simulink model "lab2_1"  (R2025b)
settings: Solver=VariableStepAuto  StartTime=0.0  StopTime=25.0  RelTol=1e-3
settings Model: Creator=mizula  LastModifiedBy=mizula

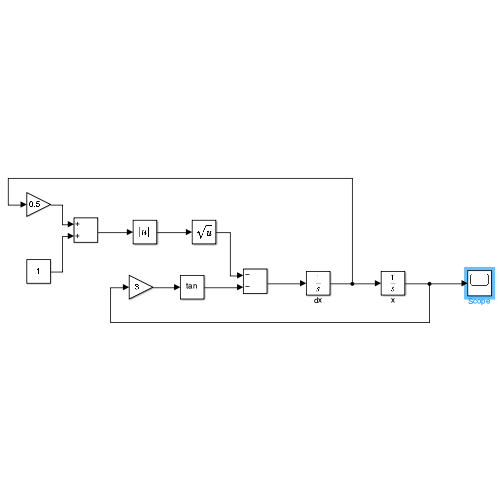
[thumbnail: Simulink's stored preview of the top-level diagram]
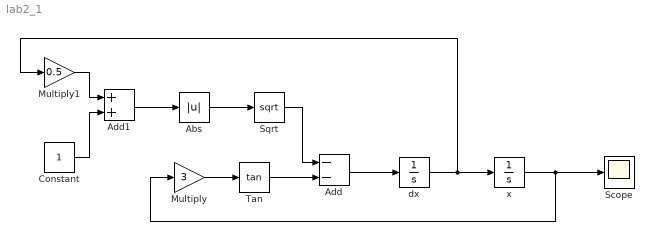
== system lab2_1 ==
  Abs : Abs  SaturateOnIntegerOverflow=off
  Add : Sum  Inputs=--
  Add1 : Sum
  Constant : Constant
  Multiply : Gain  Gain=3
  Multiply1 : Gain  Gain=0.5
  Scope : Scope
      settings: ActiveDisplayYMinimum=0.14682520044957187  ActiveDisplayYMaximum=1.5964464748927831
  Sqrt : Sqrt
  Tan : Trigonometry  Operator=tan
  dx : Integrator
  x : Integrator  InitialCondition=1
  wires:
  Add/1 -> dx/1
  dx/1 -> Multiply1/1, x/1
  Tan/1 -> Add/2
  Multiply/1 -> Tan/1
  x/1 -> Multiply/1, Scope/1
  Sqrt/1 -> Add/1
  Abs/1 -> Sqrt/1
  Add1/1 -> Abs/1
  Constant/1 -> Add1/2
  Multiply1/1 -> Add1/1
